simulink model "VMO_onlineGP_triggerTime"  (Simulink 10.3)
settings: Solver=VariableStepAuto  StartTime=0.0  StopTime=50  FixedStep=0.01  RelTol=1e-3
model workspace (MAT data in the model file):
  lambda = 0.0016
  po : num (value not decoded)
undefined symbols (not defined in the file or in its folder): mergepose
undefined symbols (not defined in the file): Pinhole
libraries: simlib_vpc_basic x6, simlib_vpc_coremath x3, simlib_vpc_gp x2
settings Model: Creator=marco  LastModifiedBy=marco  MultithreadedSim=on
settings DataIOCC: SaveFormat=Dataset  SignalLoggingSaveFormat=Dataset  ReturnWorkspaceOutputs=on
settings OptimizationCC: ExpressionDepthLimit=128  LifeSpan=auto
settings DebuggingCC: AlgebraicLoopMsg=none  UnderspecifiedInitializationDetection=Simplified  MergeDetectMultiDrivingBlocksExec=error  FcnCallInpInsideContextMsg=error  StateNameClashWarn=none  SFUnexpectedBacktrackingDiag=error  SFNoUnconditionalDefaultTransitionDiag=error  SFExecutionAtInitializationDiag=warning  ArithmeticOperatorsInVariantConditions=error
settings HardwareCC: ProdBitPerPointer=64  ProdBitPerSizeT=64  ProdBitPerPtrDiffT=64  ProdLargestAtomicFloat=Float  ProdIntDivRoundTo=Zero  ProdEndianess=LittleEndian  ProdWordSize=64  ProdHWDeviceType=Intel->x86-64 (Windows64)
settings ModelReferenceCC: PropagateSignalLabelsOutOfModel=on
settings SFSimCC: SimUseLocalCustomCode=on  CustomCodeUndefinedFunction=FilterOut
settings RTWCC: RTWUseLocalCustomCode=on  Toolchain=Clang v3.1 | gmake (64-bit Mac)
settings CodeAppCC: StateflowObjectComments=off
settings GRTTargetCC: TargetLangStandard=C99 (ISO)  CombineOutputUpdateFcns=on  GRTInterface=off
settings ConfigComp: CovMetricSettings=dwe  CovSaveCumulativeToWorkspaceVar=off  CovSaveSingleToWorkspaceVar=off  CovExternalEMLEnable=on

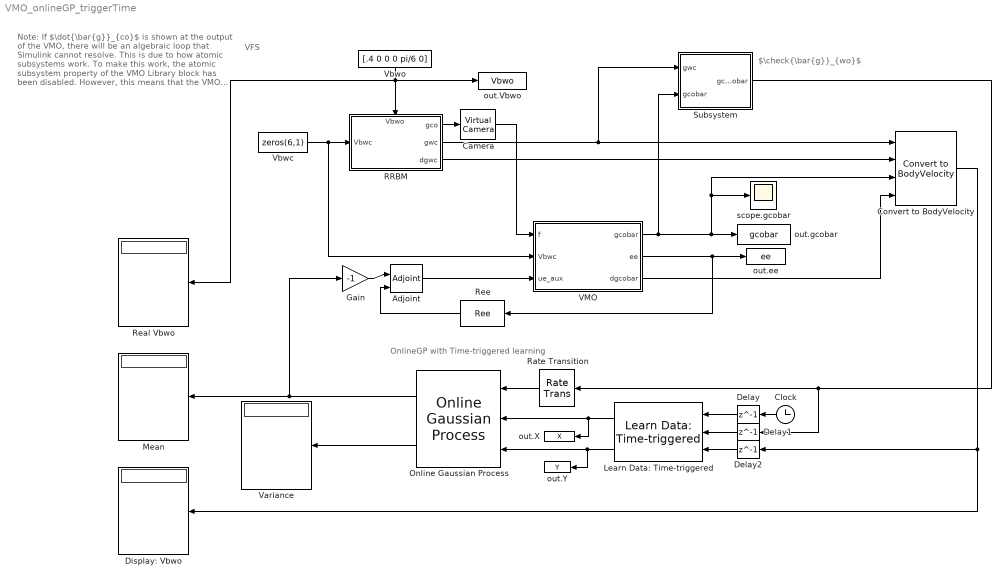
== system VMO_onlineGP_triggerTime ==
  note: OnlineGP with Time-triggered learning
  note: Note:
      | If $\dot{\bar{g}}_{co}$ is shown at the output of the VMO, there will be an algebraic loop that Simulink cannot resolve. This is due to how atomic subsystems work.
      |
      | To make this work, the atomic subsystem property of the VMO Library block has been disabled. However, this means that the VMO block in this Simulink file is unique and does NOT belong to the library. Please note that changes in the library for the VMO block therefore do not affect this simulink file, and have to be made manually!
  note: VFS
  note: $\check{\bar{g}}_{wo}$
  Adjoint : simlib_vpc_basic/Adjoint  adjointtype=orientation
      settings: SourceProductName=VPC Library
  Camera : simlib_vpc_basic/Virtual Camera  camtype=Pinhole  po=po  lambda=lambda
      settings: SourceProductName=VPC Library
  Clock : Clock
  Convert to BodyVelocity : simlib_vpc_coremath/Convert to BodyVelocity
      settings: SourceProductName=VPC Library
  Delay : Delay  DelayLength=1
  Delay1 : Delay  DelayLength=1  InitialCondition=zeros(6,1)
  Delay2 : Delay  DelayLength=1  InitialCondition=zeros(6,1)
  Display: Vbwo : Display
  Gain : Gain  Gain=-1
  Learn Data: Time-triggered : simlib_vpc_gp/Learn Data: Time-triggered  ts=0.01  T=1  M=10  forget_type=oldest
      settings: SourceProductName=VPC Library
  Mean : Display
  Online Gaussian Process : simlib_vpc_gp/Online Gaussian Process  sn_source=internal  sn=1e-2.*ones(6,1)  kernel=Squared Exponential ARD  hyp_source=internal  hyp=[5811173401.07743,21588555449944.6,1,8110042.13413100,7904.61094638263,7904.61094640294,0.200026025926779;60.7489924638542,524.808810512054,1,1.61563170712922,1.71239559901261,1.71239559901241,5.61320776710465e-12;1489.26961783243,49.4500876144320,1,0.324984946298690,0.226613543570055,0.226613543570214,1.82535781762732e-12;0.155449650516185,65.1816809298117,1,38.3822907611281,127.663031081991,127.663031082079,1.99651276292628e-06;128404403992.719,7471024903.20162,1,84140203.5908082,50182603.3525114,50182603.3525587,0.523611111558223;37.3372791443734,0.609451645130079,1,112.088235919108,638.746459440934,638.746459442022,3.48460802714492e-08]
      settings: SourceProductName=VPC Library
  RRBM : Subsystem
      settings: PortSchema="{\"entries\":[{\"content\":{\"sides\":[{\"content\":{\"connectorIds\":[\"In1\"]},\"type\":\"ConnectorPlacement.EquallySpacedRectSide\",\"uuid\":\"ce1006a6-ff18-4db7-ad69-3a60144a672f\"},{\"content\":{\"connectorIds\":[\"Out1\",\"Out2\",\"Out3\"],\"side\":\"RIGHT\"},\"type\":\"ConnectorPlacement.EquallySpacedRectSide\",\"uuid\":\"9f6b7cf2-eb23-4db0-862a-f9244538bf77\"},{\"content\":{\"connectorIds\":[\"In2\"],\"side\":\"TOP\"},\"type\":\"ConnectorPlacement.EquallySpacedRectSide\",\"uuid\":\"e4abfdaf-0145-4439-9abb-46234dad4713\"},{\"content\":{\"connectorIds\":[],\"side\":\"HIDDEN\"},\"type\":\"ConnectorPlacement.EquallySpacedRectSide\",\"uuid\":\"77f0040d-d5e2-4b47-95e1-996605172696\"}]},\"type\":\"ConnectorPlacement.EquallySpacedConnector\",\"uuid\":\"a30e6cf8-5cfd-45cc-9c7f-0b16cc268ba1\"}],\"packageUris\":[\"http://schema.mathworks.com/mf0/Connector/R2020b\"],\"version\":\"1.0\"}"
      mask Display:
      | % Glitch in Matlab: If you define a line whose starting point and end point
      | % is equal, then the entire mask block is plotted in bold
      | plot([0,0],[0,0])
      | 
      | % Draw Box
      | plot([0,1,1,0,0],[0,0,1,1,0])
      | 
      | % Write label
      | fprintf('1 Agent\n1 Target','texmode','on')
      | 
      | % Label ports
      | port_label('input',1,'V^{b}_{wc}','texmode','on')
      | port_label('input',2,'V^{b}_{wo}','texmode','on')
      | port_label('output',1,'g_{co}','texmode','on')
      | port_label('output',2,'g_{wc}','texmode','on')
      | port_label('output',3,'dg_{wc}','texmode','on')
  Rate Transition : RateTransition  OutPortSampleTime=0.01
  Real Vbwo : Display
  Ree : simlib_vpc_coremath/Ree
      settings: SourceProductName=VPC Library
  Subsystem : Subsystem
      mask Display:
      | % Write label
      | % disp('Trans','texmode','on')
      | 
      | % Label ports
      | port_label('input',1,'g_{wc}','texmode','on')
      | port_label('input',2,'g_{co,bar}','texmode','on')
      | port_label('output',1,'g^{\upsilon}_{wo,bar}','texmode','on')
  VMO : Subsystem  mask(Visual Motion Observer [V1]){gcobar0=[eye(4,3), ones(4,1)], projection=on, Ke_source=internal, Ke=5*eye(6), show_ue_aux=on, show_ee=on, show_dgcobar=on, camtype=Pinhole, fo=po, lambda=lambda}
      mask prompts: gcobar0 "Initial estimate gco_bar(0):"; projection "Use projection"; Ke_source "Observer gain source:"; Ke "Observer gain Ke"; show_ue_aux "Show feed-forward ue input"; show_ee "Show estimation error output"; show_dgcobar "Show estimation derivative"; camtype "Camera type"; fo "Feature point position coordinates (fixed in object frame Σo) [m]"; lambda "Camera focal length λ [m]"
      mask help:
      | Visual Motion Observer Block.
      | Check parameters carefully.
      mask init:
      | % Blocks
      | ueblock = find_system(gcb,'SearchDepth','1','LookUnderMasks','on',...
      |     'FollowLinks','on','Name','ue_aux');
      | 
      | if show_ue_aux && isempty(ueblock) % Show ue inport
      |     % Delete line
      |     delete_line(gcb,'Gain/1','Gain_ue/1')
      |     % Add block
      |     port_number = 3;
      |     if Ke_source == 1 % Internal
      |         port_number = 3;
      |     else % External
      |         port_number = 4;
      |     end
      |     add_block('built-in/Inport',[gcb,'/ue_aux'],'Position',[155 278 185 292],'Port',num2str(port_number));
      |     add_block('built-in/sum',[gcb,'/sum_ue'],'Position',[215 275 235 295],'Inputs','|++');
      |     % Connect lines
      |     add_line(gcb,'ue_aux/1','sum_ue/1','autorouting','smart');
      |     add_line(gcb,'sum_ue/1','Gain_ue/1','autorouting','smart');
      |     add_line(gcb,'Gain/1','sum_ue/2','autorouting','smart')
      | elseif ~show_ue_aux && ~isempty(ueblock) % Hide ue inport
      |     sum_ue = find_system(gcb,'SearchDepth','1','LookUnderMasks','on',...
      |         'FollowLinks','on','Name','sum_ue');
      |     % Delete lines
      |     delete_line(gcb,'ue_aux/1','sum_ue/1')
      |     delete_line(gcb,'sum_ue/1','Gain_ue/1')
      |     delete_line(gcb,'Gain/1','sum_ue/2')
      |     % Delete block
      |     delete_block(ueblock);
      |     delete_block(sum_ue);
      |     % Add line
      |     add_line(gcb,'Gain/1','Gain_ue/1','autorouting','smart')
      | end
      | 
      | out_port = 2;
      | 
      | % Show ee output
      | if show_ee
      |     % Add block & lines
      |     try; add_block('built-in/Outport',[gcb,'/ee'],'Port',num2str(out_port),'Position',[790 258 820 272]); end;
      |     try; add_line(gcb,'Image Jacobian/1','ee/1','autorouting','smart'); end;
      |     out_port = out_port+1;
      | else
      |     % Delete block & lines
      |     eeblock = find_system(gcb,'SearchDepth','1','LookUnderMasks','on',...
      |         'FollowLinks','on','Name','ee');
      |     try; delete_line(gcb,'Image Jacobian/1','ee/1'); end;
      |     try; delete_block(eeblock); end;
      | end
      | 
      | % Show estimation derivative dgcobar output
      | if show_dgcobar
      |     % Pass argument to rrbm block
      |     set_param([gcb,'/rrbm'],'show_dgco','on')
      |     % Add block & lines
      |     try; add_block('built-in/Outport',[gcb,'/dgcobar'],'Port',num2str(out_port),'Position',[505 333 535 347]); end;
      |     try; add_line(gcb,'rrbm/2','dgcobar/1','autorouting','smart'); end;
      | else
      |     % Delete block & lines
      |     dgcobarblock = find_system(gcb,'SearchDepth','1','LookUnderMasks','on',...
      |         'FollowLinks','on','Name','dgcobar');
      |     try; delete_line(gcb,'rrbm/2','dgcobar/1'); end;
      |     try; delete_block(dgcobarblock); end;
      |     % Pass argument to rrbm block
      |     set_param([gcb,'/rrbm'],'show_dgco','off')
      | end
      | 
      | 
      | % Switch Ke: external <-> internal
      | switch Ke_source
      |     case 1 % Make internal
      |         % Delete block & lines
      |         Ke_inport = find_system(gcb,'SearchDepth','1','LookUnderMasks','on',...
      |             'FollowLinks','on','Name','Ke_inport');
      |         Ke_mult = find_system(gcb,'SearchDepth','1','LookUnderMasks','on',...
      |             'FollowLinks','on','Name','Ke_mult');
      |         try; delete_line(gcb,'Image Jacobian/1','Ke_mult/2'); end;
      |         try; delete_line(gcb,'Ke_inport/1','Ke_mult/1'); end;
      |         try; delete_line(gcb,'Ke_mult/1','Gain/1'); end;
      |         try; delete_block(Ke_mult); end;
      |         try; delete_block(Ke_inport); end;
      | 
      |         % Add block & lines
      |         try; add_block('built-in/Gain',[gcb,'/Ke_gain'],'Gain','Ke','Multiplication','Matrix(K*u) (u vector)','Position',[415 347 490 423],'Orientation','left'); end;
      |         try; add_line(gcb,'Image Jacobian/1','Ke_gain/1','autorouting','smart'); end;
      |         try; add_line(gcb,'Ke_gain/1','Gain/1','autorouting','smart'); end;
      |     case 2 % Make external
      |         % Delete block & lines
      |         Ke_gain = find_system(gcb,'SearchDepth','1','LookUnderMasks','on',...
      |             'FollowLinks','on','Name','Ke_gain');
      |         try; delete_line(gcb,'Image Jacobian/1','Ke_gain/1'); end;
      |         try; delete_line(gcb,'Ke_gain/1','Gain/1'); end;
      |         try; delete_block(Ke_gain); end;
      | 
      |         % Add block & lines
      |         try; add_block('built-in/Inport',[gcb,'/Ke_inport'],'Position',[490 363 520 377],'Port','3','Orientation','left'); end;
      |         try; add_block('built-in/Product',[gcb,'/Ke_mult'],'Multiplication','Matrix(*)','Position',[405 359 450 406],'Orientation','left'); end;
      |         try; add_line(gcb,'Ke_inport/1','Ke_mult/1','autorouting','smart'); end;
      |         try; add_line(gcb,'Image Jacobian/1','Ke_mult/2','autorouting','smart'); end;
      |         try; add_line(gcb,'Ke_mult/1','Gain/1','autorouting','smart'); end;
      | end
      settings: MinAlgLoopOccurrences=on
      mask Help:
      | Refer to:
      | T. Hatanaka, N. Chopra, M. Fujita, and M. W. Spong, <i>Passivity-based Control and Estimation in Networked Robotics</i>, ser. Communications and Control Engineering. Springer, 2015.
      mask TypeOptions gcobar0: rrbm/gco0
      mask TypeOptions projection: rrbm/projection
      mask TypeOptions Ke_source: internal | external
      mask Callback Ke_source:
      | Ke_source = get_param(gcb,'Ke_source');
      | 
      | idx = find(strcmp(get_param(gcb,'MaskNames'),'Ke'));
      | maskvis = get_param(gcb,'MaskVisibilities');
      | switch Ke_source
      |     case 'internal' % Show Ke field
      |         maskvis{idx} = 'on';
      |     case 'external' % Hide Ke field
      |         maskvis{idx} = 'off';
      | end
      | set_param(gcb,'MaskVisibilities',maskvis);
      mask TypeOptions camtype: Virtual Camera/camtype
      mask DialogControl show_ue_aux Tooltip: If on, the internal observer input is calculated as: ue = -Ke*ee + ue_aux. The last term represents the feed-forward input, which is necessary if e.g. a GP model is used.
      mask DialogControl show_dgcobar Tooltip: If on, the estimation derivative dgcobar will be shown on the output.
      mask Display:
      | % Glitch in Matlab: If you define a line whose starting point and end point
      | % is equal, then the entire mask block is plotted in bold
      | plot([0,0],[0,0])
      | 
      | % Draw Box
      | plot([0,1,1,0,0],[0,0,1,1,0])
      | 
      | % Write label
      | % disp('VMO','texmode','on')
      | p=get_param(gcb,'Position');
      | size = min(p(3:4)-p(1:2));
      | blkscale = abs((p(3)-p(1)) / (p(4)-p(2)));
      | if abs((p(3)-p(1))) > abs((p(4)-p(2))) % block is horizontal
      |     scale = .8*[1/blkscale 1];
      | else % block is vertical
      |     scale = .8*[1 blkscale];
      | end
      | pos = [1-scale(1) 1-scale(2)]./2;
      | image('ico_vmo.png',[pos scale],'off')
      | 
      | % Label input ports
      | port_label('input',1,'f','texmode','on')
      | port_label('input',2,'V^{b}_{wc}','texmode','on')
      | Ke_source = get_param(gcb, 'Ke_source');
      | port_number = 3;
      | switch Ke_source
      |     case 'internal'
      |     case 'external'
      |         port_label('input',3,'K_e','texmode','on')
      |         port_number = 4;
      | end
      | show_ue_aux = get_param(gcb, 'show_ue_aux');
      | if show_ue_aux == "on"
      |     port_label('input',port_number,'u_{e,aux}','texmode','on')
      | end
      | 
      | % Label output ports
      | port_label('output',1,'g_{co,bar}','texmode','on')
      | port_number = 2;
      | show_ee = get_param(gcb, 'show_ee');
      | if show_ee == "on"
      |     port_label('output',port_number,'e_{e}','texmode','on')
      |     port_number = port_number+1;
      | end
      | show_dgcobar = get_param(gcb, 'show_dgcobar');
      | if show_dgcobar == "on"
      |     port_label('output',port_number,'dg_{co,bar}','texmode','on')
      |     port_number = port_number+1;
      | end
  Variance : Display
  Vbwc : Constant  Value=zeros(6,1)
  Vbwo : Constant  Value=[.4 0 0 0 pi/6 0]
  out.Vbwo : ToWorkspace  VariableName=Vbwo  SaveFormat=Structure With Time  SampleTime=-1
  out.X : ToWorkspace  VariableName=X  SaveFormat=Structure With Time  SampleTime=-1
  out.Y : ToWorkspace  VariableName=Y  SaveFormat=Structure With Time  SampleTime=-1
  out.ee : ToWorkspace  VariableName=ee  SaveFormat=Structure With Time  SampleTime=-1
  out.gcobar : ToWorkspace  VariableName=gcobar  SaveFormat=Structure With Time  SampleTime=-1
  scope.gcobar : Scope
  wires:
  Vbwc/1 -> VMO/2(Vbwc), RRBM/1(Vbwc)
  Vbwo/1 -> RRBM/2(Vbwo), Real Vbwo/1, out.Vbwo/1
  RRBM/1(gco) -> Camera/1
  VMO/2(ee) -> Ree/1, out.ee/1
  Camera/1 -> VMO/1(f)
  VMO/1(gcobar) -> out.gcobar/1, scope.gcobar/1, Convert to BodyVelocity/3, Subsystem/2(gcobar)
  Online Gaussian Process/2 -> Variance/1
  Gain/1 -> Adjoint/1
  Adjoint/1 -> VMO/3(ue_aux)
  Ree/1 -> Adjoint/2
  RRBM/2(gwc) -> Convert to BodyVelocity/1, Subsystem/1(gwc)
  Subsystem/1(gcheck_wobar) -> Rate Transition/1, Delay1/1
  Clock/1 -> Delay/1
  Learn Data: Time-triggered/1 -> out.X/1, Online Gaussian Process/2
  Learn Data: Time-triggered/2 -> out.Y/1, Online Gaussian Process/3
  Online Gaussian Process/1 -> Mean/1, Gain/1
  Rate Transition/1 -> Online Gaussian Process/1
  VMO/3(dgcobar) -> Convert to BodyVelocity/4
  Convert to BodyVelocity/1 -> Display: Vbwo/1, Delay2/1
  RRBM/3(dgwc) -> Convert to BodyVelocity/2
  Delay/1 -> Learn Data: Time-triggered/1
  Delay1/1 -> Learn Data: Time-triggered/2
  Delay2/1 -> Learn Data: Time-triggered/3

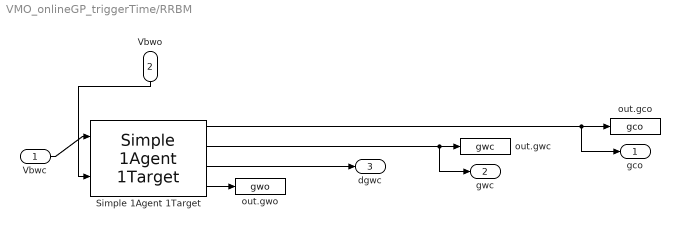
== system VMO_onlineGP_triggerTime/RRBM ==
  Vbwc : Inport
  Vbwo : Inport  Port=2
  Simple 1Agent 1Target : simlib_vpc_basic/Simple 1Agent 1Target  gwc0=mergepose(rotx(-90),[0; -5; 0])  projectionAgent=on  gwo0=mergepose(rotx(-90),[0.3; 0.1; 0.1])  projectionTarget=on  showgwc=on  showdgwc=on  showgwo=on  showdgwo=off
      settings: SourceProductName=VPC Library
  out.gco : ToWorkspace  VariableName=gco  SaveFormat=Structure With Time  SampleTime=-1
  out.gwc : ToWorkspace  VariableName=gwc  SaveFormat=Structure With Time  SampleTime=-1
  out.gwo : ToWorkspace  VariableName=gwo  SaveFormat=Structure With Time  SampleTime=-1
  gco : Outport
  gwc : Outport  Port=2
  dgwc : Outport  Port=3
  wires:
  Vbwo/1 -> Simple 1Agent 1Target/2
  Vbwc/1 -> Simple 1Agent 1Target/1
  Simple 1Agent 1Target/2 -> gwc/1, out.gwc/1
  Simple 1Agent 1Target/4 -> out.gwo/1
  Simple 1Agent 1Target/1 -> gco/1, out.gco/1
  Simple 1Agent 1Target/3 -> dgwc/1

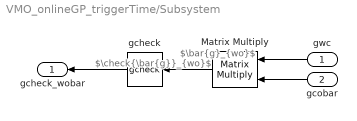
== system VMO_onlineGP_triggerTime/Subsystem ==
  note: $\bar{g}_{wo}$
  note: $\check{\bar{g}}_{wo}$
  gwc : Inport
  gcobar : Inport  Port=2
  Matrix Multiply : Product  Multiplication=Matrix(*)
  gcheck : simlib_vpc_coremath/gcheck
      settings: SourceProductName=VPC Library
  gcheck_wobar : Outport
  wires:
  gwc/1 -> Matrix Multiply/1
  gcobar/1 -> Matrix Multiply/2
  gcheck/1 -> gcheck_wobar/1
  Matrix Multiply/1 -> gcheck/1

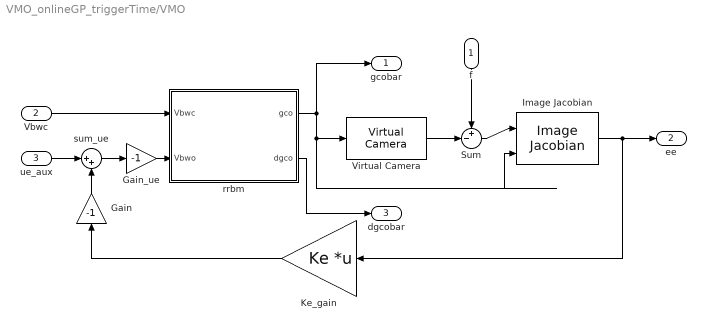
== system VMO_onlineGP_triggerTime/VMO ==
  f : Inport
  Vbwc : Inport  Port=2
  ue_aux : Inport  Port=3
  Gain : Gain  Gain=-1
  Gain_ue : Gain  Gain=-1
  Image Jacobian : simlib_vpc_basic/Image Jacobian  po=fo  lambda=lambda
      settings: SourceProductName=VPC Library
  Ke_gain : Gain  Gain=Ke  Multiplication=Matrix(K*u) (u vector)
  Sum : Sum  Inputs=+-|
  Virtual Camera : simlib_vpc_basic/Virtual Camera  camtype=Pinhole  po=fo  lambda=lambda
      settings: SourceProductName=VPC Library
  rrbm : Subsystem  mask(Relative Rigid Body Motion Block [V1]){gco0=gcobar0, projection=on, show_dgco=on}
      mask prompts: gco0 "Initial condition gco(0):"; projection "Use projection"; show_dgco "Show dgco"
      mask help: Relative rigid body motion of agent A as it can be observed from agent B.
      mask init:
      | block = find_system(gcb,'LookUnderMasks','on',...
      |     'FollowLinks','on','Name','Projection');
      | 
      | if projection && isempty(block) % Turn on projection
      |     % Delete lines
      |     delete_line(gcb,'Integrator/1','gco/1')
      |     delete_line(gcb,'Integrator/1','rrbm/3')
      |     
      |     % Add block
      |     add_block([bdroot(gcb),'/Projection'],[gcb,'/Projection'],'inputtype','pose');
      |     
      |     % Connect lines
      |     add_line(gcb,'Integrator/1','Projection/1','autorouting','smart')
      |     add_line(gcb,'Projection/1','gco/1','autorouting','smart')
      |     add_line(gcb,'Projection/1','rrbm/3','autorouting','smart')
      | elseif ~projection && ~isempty(block) % Turn off projection
      |     % Delete lines
      |     delete_line(gcb,'Integrator/1','Projection/1')
      |     delete_line(gcb,'Projection/1','gco/1')
      |     delete_line(gcb,'Projection/1','rrbm/3')
      | 
      |     % Delete block
      |     delete_block(block);
      | 
      |     % Connect blocks
      |     add_line(gcb,'Integrator/1','gco/1','autorouting','smart')
      |     add_line(gcb,'Integrator/1','rrbm/3','autorouting','smart')
      | end
      | 
      | % Show dgco output
      | if show_dgco
      |     % Add block & lines
      |     try; add_block('built-in/Outport',[gcb,'/dgco'],'Port','2','Position',[510 193 540 207]); end;
      |     try; add_line(gcb,'rrbm/1','dgco/1','autorouting','smart'); end;
      | else
      |     % Delete block & lines
      |     dgcoblock = find_system(gcb,'SearchDepth','1','LookUnderMasks','on',...
      |         'FollowLinks','on','Name','dgco');
      |     try; delete_line(gcb,'rrbm/1','dgco/1'); end;
      |     try; delete_block(dgcoblock); end;
      | end
      settings: MinAlgLoopOccurrences=on
      mask Help:
      | Refer to:
      | T. Hatanaka, N. Chopra, M. Fujita, and M. W. Spong, <i>Passivity-based Control and Estimation in Networked Robotics</i>, ser. Communications and Control Engineering. Springer, 2015.
      mask TypeOptions gco0: Integrator/InitialCondition
      mask DialogControl show_dgco Tooltip: If on, the internal state derivative of gco will be shown as an output
      mask Display:
      | % Glitch in Matlab: If you define a line whose starting point and end point
      | % is equal, then the entire mask block is plotted in bold
      | plot([0,0],[0,0])
      | 
      | % Draw Box
      | plot([0,1,1,0,0],[0,0,1,1,0])
      | 
      | % Write label
      | fprintf('Relative Rigid\nBody Motion','texmode','on')
      | 
      | % Label ports
      | port_label('input',1,'V^{b}_{wc}','texmode','on')
      | port_label('input',2,'V^{b}_{wo}','texmode','on')
      | port_label('output',1,'g_{co}','texmode','on')
      | if strcmp(get_param(gcb,'show_dgco'),'on')
      |     port_label('output',2,'dg_{co}','texmode','on')
      | end
  sum_ue : Sum  Inputs=|++
  gcobar : Outport
  ee : Outport  Port=2
  dgcobar : Outport  Port=3
  wires:
  Ke_gain/1 -> Gain/1
  Image Jacobian/1 -> Ke_gain/1, ee/1
  Gain_ue/1 -> rrbm/2(Vbwo)
  Vbwc/1 -> rrbm/1(Vbwc)
  f/1 -> Sum/1
  Sum/1 -> Image Jacobian/1
  rrbm/1(gco) -> Virtual Camera/1, Image Jacobian/2, gcobar/1
  Virtual Camera/1 -> Sum/2
  ue_aux/1 -> sum_ue/1
  sum_ue/1 -> Gain_ue/1
  Gain/1 -> sum_ue/2
  rrbm/2(dgco) -> dgcobar/1

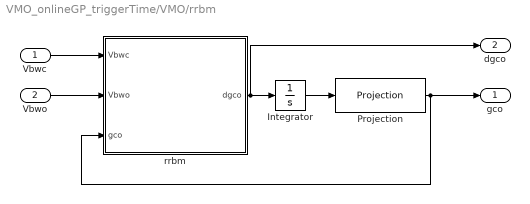
== system VMO_onlineGP_triggerTime/VMO/rrbm ==
  Vbwc : Inport
  Vbwo : Inport  Port=2
  Integrator : Integrator  InitialCondition=gco0
  Projection : simlib_vpc_basic/Projection  projectiontype=averaging  inputtype=pose
      settings: SourceProductName=VPC Library
  rrbm : MATLAB Function  TreatAsAtomicUnit=on
  gco : Outport
  dgco : Outport  Port=2
  wires:
  Vbwc/1 -> rrbm/1(Vbwc)
  rrbm/1(dgco) -> Integrator/1, dgco/1
  Vbwo/1 -> rrbm/2(Vbwo)
  Integrator/1 -> Projection/1
  Projection/1 -> gco/1, rrbm/3(gco)

== matlab function VMO/rrbm/rrbm ==
  data: Vbwc input double size=6; Vbwo input double size=6; dgco output double size=[4,4]; gco input double size=[4,4]
function dgco = slx_rrbm(Vbwc,Vbwo,gco) %#codegen
% Function Wrapper
%
% Editor:
%   OMAINSKA Marco - Doctoral Student, Cybernetics
%       <marcoomainska@g.ecc.u-tokyo.ac.jp>
% Review:
%   YAMAUCHI Junya - Assistant Professor
%       <junya_yamauchi@ipc.i.u-tokyo.ac.jp>
%
% Property of: Fujita-Yamauchi Lab, University of Tokyo, 2021
% e-mail: marcoomainska@g.ecc.u-tokyo.ac.jp
% Website: https://www.scl.ipc.i.u-tokyo.ac.jp
% March 2021, Last modified: 2021-MAR-08
%
%------------- BEGIN CODE --------------

% "rrbm" is a MATLAB function on the MATLAB path
dgco = rrbm(Vbwc, Vbwo, gco);

%------------- END CODE --------------
end
